simulink model "BotModell2"  (R2024a)
settings: Solver=VariableStepAuto  StartTime=0.0  StopTime=2  RelTol=1e-3
values from neighbouring files (symbols this model uses):
  A = zeros(n, n)    [Model1numericalPSA.m]    (also in MotorSens2.m = A_func(x0s,u0,p_sym,z0); Parameter.m = A_func(x0s,u0,z0); ParamsModell2.m = A_func(x0s,u0,z0); Sensitivitaetsanalyse.m = A_func(x0s,u0,z0))
  b = b_func(x0s,u0,p_sym,z0)    [MotorSens2.m]    (also in Parameter.m = b_func(x0s,u0,z0); ParamsModell2.m = b_func(x0s,u0,z0); Sensitivitaetsanalyse.m = b_func(x0s,u0,z0))
  c = c_func(x0s,u0,p_sym,z0)    [MotorSens2.m]    (also in Parameter.m = c_func(x0s,u0,z0); ParamsModell2.m = c_func(x0s,u0,z0); Sensitivitaetsanalyse.m = c_func(x0s,u0,z0))
libraries: mobileRoboticsLib x1
settings Model: Creator=jakob  LastModifiedBy=jakob

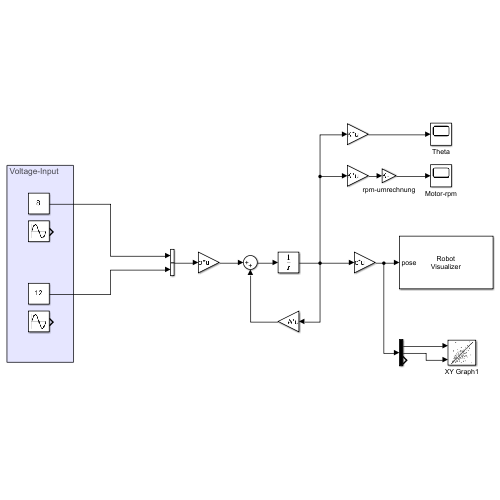
[thumbnail: Simulink's stored preview of the top-level diagram]
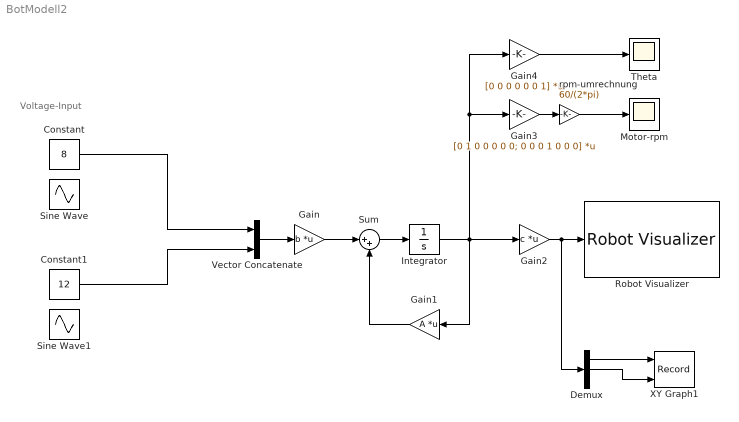
== system BotModell2 ==
  note: Voltage-Input
  Constant : Constant  Value=8  SampleTime=1
  Constant1 : Constant  Value=12  SampleTime=1
  Demux : Demux  Outputs=3
  Gain : Gain  Gain=b  Multiplication=Matrix(K*u)
  Gain1 : Gain  Gain=A  Multiplication=Matrix(K*u)
  Gain2 : Gain  Gain=c  Multiplication=Matrix(K*u)
  Gain3 : Gain  Gain=[0 1 0 0 0 0 0; 0 0 0 1 0 0 0]  Multiplication=Matrix(K*u)
  Gain4 : Gain  Gain=[0 0 0 0 0 0 1]  Multiplication=Matrix(K*u)
  Integrator : Integrator
  Motor-rpm : Scope
  Robot Visualizer : mobileRoboticsLib/Environments/Robot Visualizer  robotRadius=0.1  mapName=myMap  showTrajectory=on  hasWaypoints=off  hasLidar=off  sensorOffset=[ 0, 0 ]  scanAngles=[ -pi/4, 0, pi/4 ]  hasObjDetector=off  objDetectorOffset=[ 0, 0 ]  objDetectorAngle=0  objDetectorFOV=pi/4  objDetectorMaxRange=5  objectColors=[ 1, 0, 0; 0, 1, 0; 0, 0, 1 ]  objectMarkers=s
  Sine Wave : Sin  Amplitude=4  Bias=8  Frequency=2  SampleTime=0
  Sine Wave1 : Sin  Amplitude=2  Bias=9  Frequency=8  SampleTime=0
  Sum : Sum  Inputs=|++
  Theta : Scope
  Vector Concatenate : Concatenate
  XY Graph1 : Record  FileSettingsInternal="{\"entries\":[{\"content\":{\"excelSettings\":{\"content\":{},\"type\":\"Streamout.ExcelSettings\"}},\"type\":\"Streamout.FileSettingStorage\",\"uuid\":\"\"}],\"packageUris\":[\"http:\\/\\/schema.mathworks.com\\/mf0\\/streamout_blocks\\/R2020a\"],\"version\":\"1.0\"}"  Layout=[1 1]  SignalsInternal="{\"entries\":[{\"content\":{\"signals\":[{\"content\":{\"blockPath\":[],\"dimensions\":[1],\"domain\":\"\",\"lineColor\":\"#a2142f\",\"plots\":[ 1 ],\"port\":1,\"sid\":[\"\"],\"signalID\":1,\"signalName\":\"Demux:1\"},\"type\":\"RecordBlkView.Signal\",\"uuid\":\"\"},{\"content\":{\"blockPath\":[],\"dimensions\":[1],\"domain\":\"\",\"lineColor\":\"#139fff\",\"plots\":[ 1 ],\"port\":2,\"sid\":[\"\"],\"signalID\":2,\"signalName\":\"Demux:2\"},\"type\":\"RecordBlkView.Signal\",\"uuid\":\"\"}]},\"type\":\"RecordBlkView.InputSignals\",\"uuid\":\"\"}],\"packageUris\":[\"http:\\/\\/schema.mathworks.com\\/mf0\\/streamout_blocks\\/R2020a\"],\"version\":\"1.0\"}"  VisualizationBindings="{\"xyplotplugin\":{\"info\":[{\"series\":[{\"bindingParametersList\":[{\"parameter\":\"X-Axis\",\"signalID\":1,\"signalName\":\"Demux:1\"},{\"parameter\":\"Y-Axis\",\"signalID\":2,\"signalName\":\"Demux:2\"}],\"seriesID\":0}],\"subplotID\":1}]}}"  CompatibilityTag=XY
  rpm-umrechnung : Gain  Gain=60/(2*pi)
  wires:
  Vector Concatenate/1 -> Gain/1
  Gain/1 -> Sum/1
  Sum/1 -> Integrator/1
  Gain1/1 -> Sum/2
  Integrator/1 -> Gain2/1, Gain4/1, Gain3/1, Gain1/1
  Gain2/1 -> Demux/1, Robot Visualizer/1
  Demux/1 -> XY Graph1/1
  Demux/2 -> XY Graph1/2
  Constant/1 -> Vector Concatenate/1
  Constant1/1 -> Vector Concatenate/2
  Gain3/1 -> rpm-umrechnung/1
  rpm-umrechnung/1 -> Motor-rpm/1
  Gain4/1 -> Theta/1
